simulink library "WiggleDelayLib"  (R2022b)
settings: Solver=VariableStepAuto  StartTime=0.0  StopTime=10.0  RelTol=1e-3
undefined symbols (not defined in the file or in its folder): carModel, frame_size, mode, sample_rate_in_hertz, sysin_channel_count
libraries: FeaturePath x1, Delay x1
settings Model: Creator=jb1046154  LastModifiedBy=sa1045272
settings SolverCC: AlgebraicLoopSolver=TrustRegion
settings DebuggingCC: UnconnectedInputMsg=warning  UnconnectedOutputMsg=warning  UnconnectedLineMsg=warning  SFMachineParentedDataDiag=warning
settings ModelReferenceCC: EnableRefExpFcnMdlSchedulingChecks=on

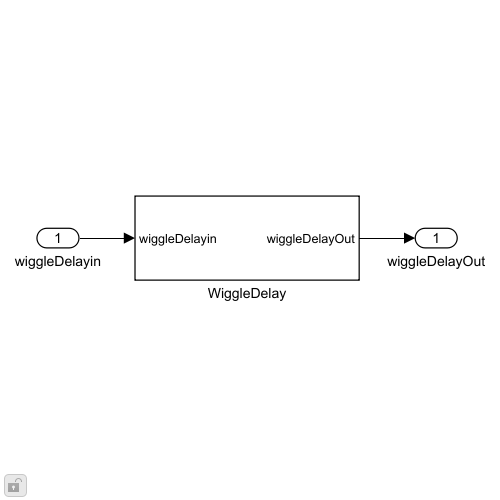
[thumbnail: Simulink's stored preview of the top-level diagram]
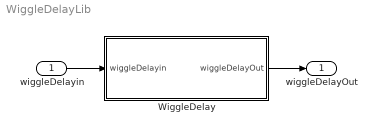
== system WiggleDelayLib ==
  wiggleDelayin : Inport  OutDataTypeStr=single  PortDimensions=[frame_size sysin_channel_count]  SampleTime=1/sample_rate_in_hertz * frame_size
  WiggleDelay : Subsystem
  wiggleDelayOut : Outport
  wires:
  WiggleDelay/1(wiggleDelayOut) -> wiggleDelayOut/1
  wiggleDelayin/1 -> WiggleDelay/1(wiggleDelayin)

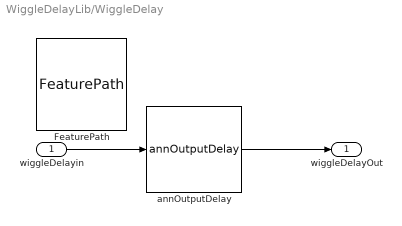
== system WiggleDelayLib/WiggleDelay ==
  wiggleDelayin : Inport  OutDataTypeStr=single
  FeaturePath : FeaturePath/FeaturePath  FeatureName=WiggleDelay_  IsGroup=off  GroupNumber=-1  DeclarePackages=off  PackageNames=mode,carModel  IsToolGroup=off  TriggerInit=[20 69 110 161]
  annOutputDelay : Delay/annOutputDelay  delay_value=wiggleDelay.delaySamples  maxdelay=wiggleDelay.maxDelaySamples
  wiggleDelayOut : Outport
  wires:
  annOutputDelay/1 -> wiggleDelayOut/1
  wiggleDelayin/1 -> annOutputDelay/1
